simulink model "motor_position_SIMULINK"  (R2021a)
settings: Solver=ode15s  StartTime=0.0  StopTime=0.08  RelTol=1e-3
values from neighbouring files (symbols this model uses):
  b = 3.5007E-6    (= 3.5007e-06)    [motor_position.m]
  J = 3.2284E-6    (= 3.2284e-06)    [motor_position.m]
  K = 0.0274    [motor_position.m]
  L = 2.75E-6    (= 2.75e-06)    [motor_position.m]
  R = 4    [motor_position.m]
settings Model: Creator=Lenovo  LastModifiedBy=Lenovo

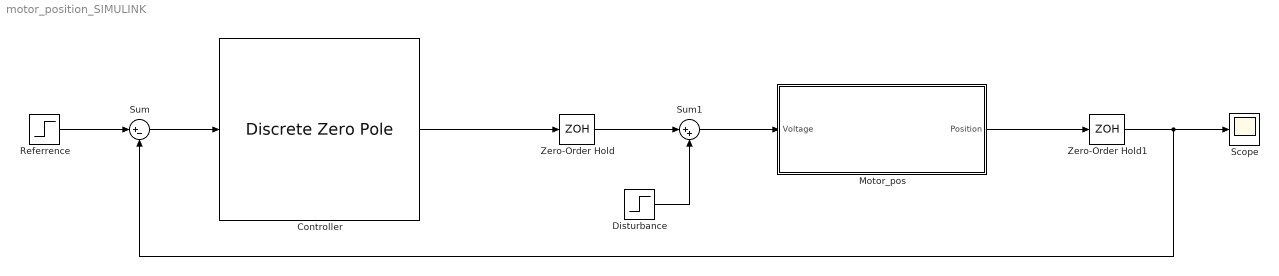
== system motor_position_SIMULINK ==
  Controller : DiscreteZeroPole  Zeros=[0.95 0.8 0.8]  Poles=[1 0.6 -0.98]  Gain=800  SampleTime=0.001
  Disturbance : Step  Time=0.03  SampleTime=0
  Motor_pos : Subsystem
  Referrence : Step  Time=0  SampleTime=0
  Scope : Scope
  Sum : Sum  Inputs=|+-
  Sum1 : Sum  Inputs=|++
  Zero-Order Hold : ZeroOrderHold  SampleTime=0.001
  Zero-Order Hold1 : ZeroOrderHold  SampleTime=0.001
  wires:
  Motor_pos/1(Position) -> Zero-Order Hold1/1
  Zero-Order Hold1/1 -> Sum/2, Scope/1
  Controller/1 -> Zero-Order Hold/1
  Referrence/1 -> Sum/1
  Sum/1 -> Controller/1
  Zero-Order Hold/1 -> Sum1/1
  Sum1/1 -> Motor_pos/1(Voltage)
  Disturbance/1 -> Sum1/2

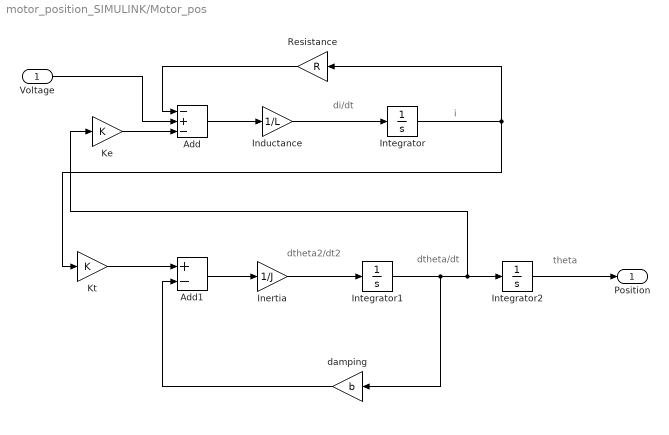
== system motor_position_SIMULINK/Motor_pos ==
  note: theta
  note: dtheta/dt
  note: dtheta2/dt2
  note: i
  note: di/dt
  Voltage : Inport
  Add : Sum  Inputs=-+-
  Add1 : Sum  Inputs=+-
  Inductance : Gain  Gain=1/L
  Inertia : Gain  Gain=1/J
  Integrator : Integrator
  Integrator1 : Integrator
  Integrator2 : Integrator
  Ke : Gain  Gain=K
  Kt : Gain  Gain=K
  Resistance : Gain  Gain=R
  damping : Gain  Gain=b
  Position : Outport
  wires:
  Add1/1 -> Inertia/1
  Integrator1/1 -> damping/1, Ke/1, Integrator2/1
  Integrator/1 -> Kt/1, Resistance/1
  damping/1 -> Add1/2
  Resistance/1 -> Add/1
  Add/1 -> Inductance/1
  Kt/1 -> Add1/1
  Inertia/1 -> Integrator1/1
  Voltage/1 -> Add/2
  Inductance/1 -> Integrator/1
  Ke/1 -> Add/3
  Integrator2/1 -> Position/1
